simulink model "SimExe2"  (R2020b)
settings: Solver=VariableStepAuto  StartTime=0.0  StopTime=tf  FixedStep=0.001  MaxStep=tf/1e4  RelTol=1e-4  AbsTol=1e-4
values from neighbouring files (symbols this model uses):
  cf = 0    [MainEs2.m]
  IC = [0,pi-pi*0.1]'    [MainEs2.m]
  Wamp = 0.1    [MainEs2.m]
undefined symbols (not defined in the file or in its folder): K
settings Model: Creator=emanuele riva  LastModifiedBy=emanuele riva
settings SolverCC: AutoScaleAbsTol=off
settings DataIOCC: ReturnWorkspaceOutputs=off
settings DebuggingCC: ArithmeticOperatorsInVariantConditions=warning
settings SFSimCC: SimUseLocalCustomCode=off  CustomCodeUndefinedFunction=UseInterfaceOnly
settings RTWCC: RTWUseLocalCustomCode=off
settings CodeAppCC: StateflowObjectComments=on

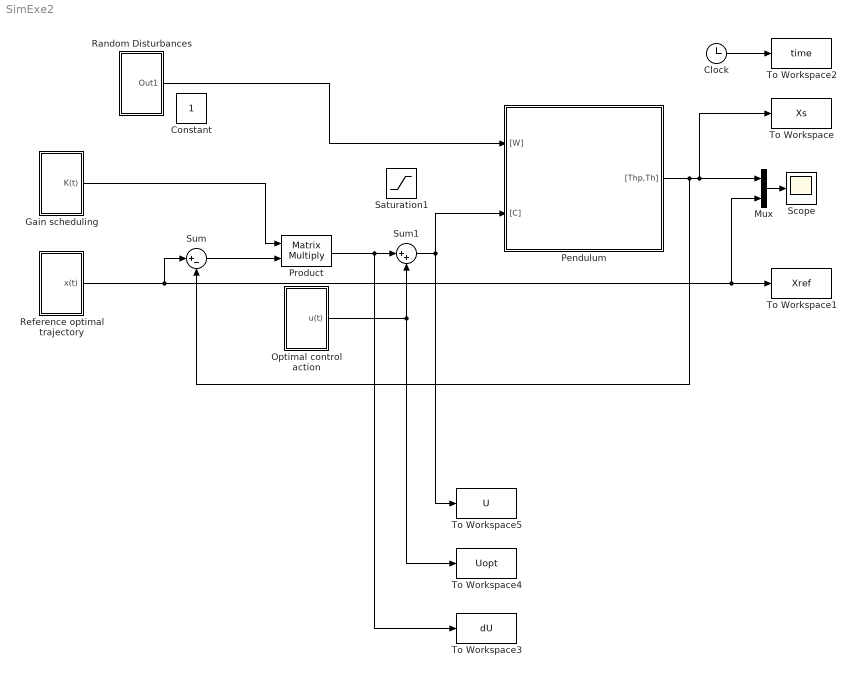
== system SimExe2 ==
  Clock : Clock
  Gain scheduling : Subsystem
  Mux : Mux  Inputs=2
  Optimal control action : Subsystem
  Pendulum : Subsystem
  Product : Product  Multiplication=Matrix(*)
  Random Disturbances : Subsystem
  Reference optimal trajectory : Subsystem
  Saturation1 : Saturate  UpperLimit=0.3  LowerLimit=-0.3
  Scope : Scope
  Sum : Sum  Inputs=|+-
  Sum1 : Sum  Inputs=|++
  To Workspace : ToWorkspace  VariableName=Xs  SaveFormat=Timeseries  SampleTime=-1
  To Workspace1 : ToWorkspace  VariableName=Xref  SaveFormat=Timeseries  SampleTime=-1
  To Workspace2 : ToWorkspace  VariableName=time  SaveFormat=Timeseries  SampleTime=-1
  To Workspace3 : ToWorkspace  VariableName=dU  SaveFormat=Timeseries  SampleTime=-1
  To Workspace4 : ToWorkspace  VariableName=Uopt  SaveFormat=Timeseries  SampleTime=-1
  To Workspace5 : ToWorkspace  VariableName=U  SaveFormat=Timeseries  SampleTime=-1
  Constant : Constant  IOType=siggen
  wires:
  Random Disturbances/1(Out1) -> Pendulum/1("[W]")
  Pendulum/1("[Thp,Th]") -> To Workspace/1, Mux/1, Sum/2
  Reference optimal trajectory/1(x(t)) -> Sum/1, To Workspace1/1, Mux/2
  Gain scheduling/1(K(t)) -> Product/1
  Product/1 -> Sum1/1, To Workspace3/1
  Optimal control action/1(u(t)) -> To Workspace4/1, Sum1/2
  Mux/1 -> Scope/1
  Clock/1 -> To Workspace2/1
  Sum/1 -> Product/2
  Sum1/1 -> Pendulum/2("[C]"), To Workspace5/1

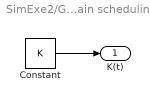
== system SimExe2/Gain scheduling ==
  Constant : Constant  Value=K  VectorParams1D=off
  K(t) : Outport
  wires:
  Constant/1 -> K(t)/1

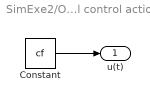
== system SimExe2/Optimal control action ==
  Constant : Constant  Value=cf
  u(t) : Outport
  wires:
  Constant/1 -> u(t)/1

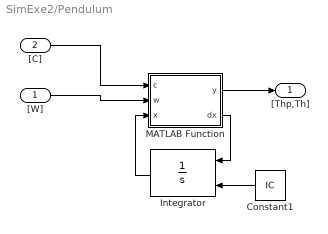
== system SimExe2/Pendulum ==
  "[W]" : Inport
  "[C]" : Inport  Port=2
  Constant1 : Constant  Value=IC
  Integrator : Integrator  InitialConditionSource=external
  MATLAB Function : MATLAB Function  TreatAsAtomicUnit=on
  "[Thp,Th]" : Outport
  wires:
  MATLAB Function/2(dx) -> Integrator/1
  Integrator/1 -> MATLAB Function/3(x)
  Constant1/1 -> Integrator/2
  MATLAB Function/1(y) -> "[Thp,Th]"/1
  "[C]"/1 -> MATLAB Function/1(c)
  "[W]"/1 -> MATLAB Function/2(w)

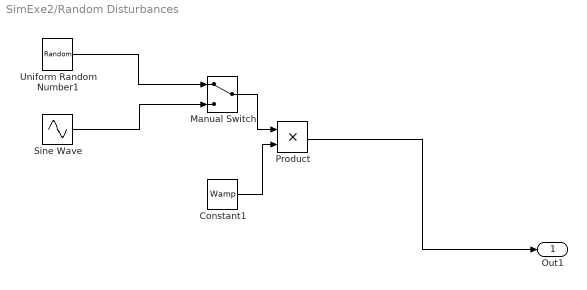
== system SimExe2/Random Disturbances ==
  Constant1 : Constant  Value=Wamp
  Manual Switch : ManualSwitch
  Product : Product
  Sine Wave : Sin  Frequency=2*pi*100  SampleTime=0
  Uniform Random Number1 : UniformRandomNumber  SampleTime=tf/1000
  Out1 : Outport
  wires:
  Product/1 -> Out1/1
  Constant1/1 -> Product/2
  Uniform Random Number1/1 -> Manual Switch/1
  Sine Wave/1 -> Manual Switch/2
  Manual Switch/1 -> Product/1

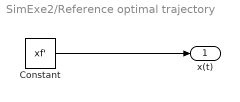
== system SimExe2/Reference optimal trajectory ==
  Constant : Constant  Value=xf'  VectorParams1D=off
  x(t) : Outport
  wires:
  Constant/1 -> x(t)/1

== matlab function SimExe2/Pendulum/MATLAB Function ==
  data: c input; w input; y output; dx output; x input
function [y,dx]  = fcn(c,w,x)

m = 1;
g = 9.81;
L = 0.1;
zeta = 0.02;
w0 = sqrt(g/L);

dx = zeros(2,1);

u = c(1) + w(1);

dx(1) = - 2*zeta*w0*x(1) - w0^2*sin(x(2)) + u/L^2/m;
dx(2) = x(1);

y = [x(1);x(2)];
